simulink model "Quantizer"  (R2023b)
settings: Solver=VariableStepAuto  StartTime=0.0  StopTime=10.0  RelTol=1e-3
libraries: simulink_extras x1
settings Model: Creator=HP  LastModifiedBy=HP

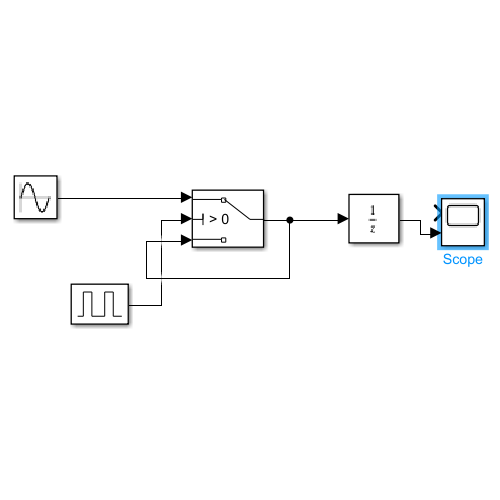
[thumbnail: Simulink's stored preview of the top-level diagram]
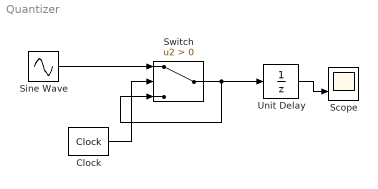
== system Quantizer ==
  Clock : simulink_extras/Flip Flops/Clock  period=0.3
  Scope : Scope  NumInputPorts=2
  Sine Wave : Sin  Amplitude=5  SampleTime=0
  Switch : Switch  Criteria=u2 > Threshold  OutMin=1  RndMeth=Zero  SaturateOnIntegerOverflow=off  InputSameDT=off
  Unit Delay : UnitDelay  SampleTime=-1  HasFrameUpgradeWarning=on
  wires:
  Sine Wave/1 -> Switch/1
  Clock/1 -> Switch/2
  Switch/1 -> Switch/3, Unit Delay/1
  Unit Delay/1 -> Scope/2
